simulink model "simulation_part1"  (R2021b)
settings: Solver=VariableStepAuto  StartTime=0.0  StopTime=10.0  RelTol=1e-3
values from neighbouring files (symbols this model uses):
  A = [0.0702214917532  -0.116010526395  -1.08987824045; 0.410067295195  -0.932250543618  -1.24586844105; -0.123091124979  1.5728866522  -0.314709957878]    [ex2_data.mat]
  B1 = [-0.999067654878  0.651260985893; 0.287497412628  0.148151711186; 0.248638319418  2.25662896165]    [ex2_data.mat]
  B2 = [0.722863093118  0.264721524509; 0.0846003934803  0.180309892623; -1.95559499489  1.07897348192]    [ex2_data.mat]
  C1 = [2.31275280612  0.189359533817  1.67949548769; 0.186530271276  1.56272046404  -1.25277472596]    [ex2_data.mat]
  C2 = [-0.336197041449  0.851608289148  0.411251123774; 1.34398190607  0.500911743536  0.482620057996]    [ex2_data.mat]
  D1 = [1  0; 0  1]    [ex2_data.mat]
  K = inv(R)*B2'*P    [ex2.m]
settings Model: Creator=Marius  LastModifiedBy=Marius

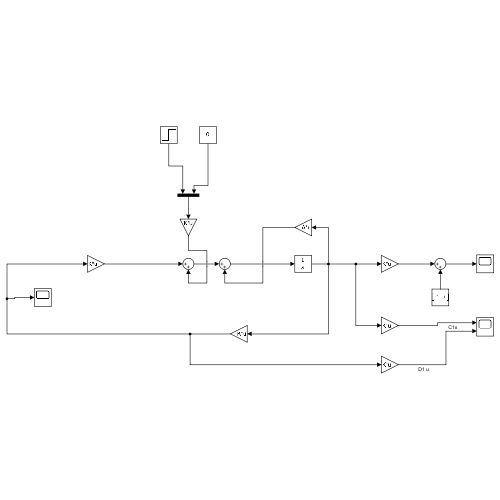
[thumbnail: Simulink's stored preview of the top-level diagram]
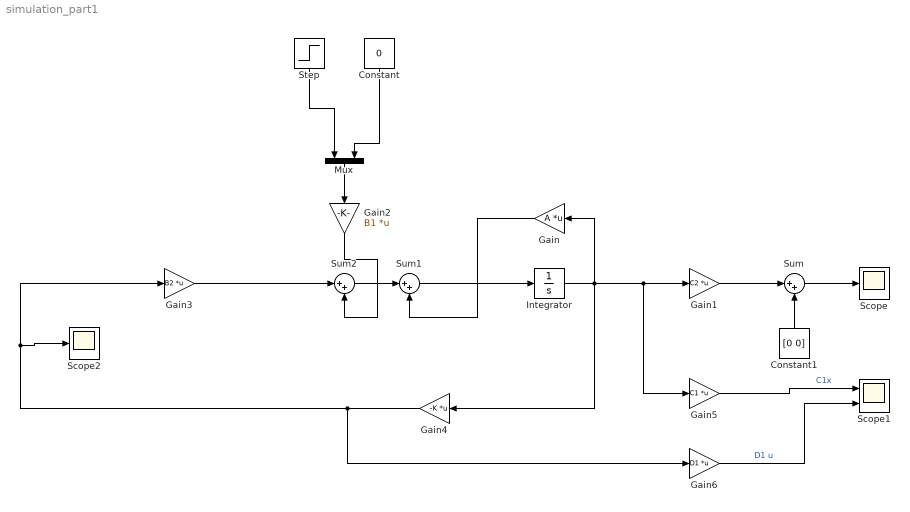
== system simulation_part1 ==
  Constant : Constant  Value=0
  Constant1 : Constant  Value=[0 0]
  Gain : Gain  Gain=A  Multiplication=Matrix(K*u)
  Gain1 : Gain  Gain=C2  Multiplication=Matrix(K*u)
  Gain2 : Gain  Gain=B1  Multiplication=Matrix(K*u)
  Gain3 : Gain  Gain=B2  Multiplication=Matrix(K*u)
  Gain4 : Gain  Gain=-K  Multiplication=Matrix(K*u)
  Gain5 : Gain  Gain=C1  Multiplication=Matrix(K*u)
  Gain6 : Gain  Gain=D1  Multiplication=Matrix(K*u)
  Integrator : Integrator
  Mux : Mux  Inputs=2
  Scope : Scope
  Scope1 : Scope  NumInputPorts=2
  Scope2 : Scope
  Step : Step  SampleTime=0
  Sum : Sum  Inputs=|++
  Sum1 : Sum  Inputs=|++
  Sum2 : Sum  Inputs=|++
  wires:
  Integrator/1 -> Gain4/1, Gain/1, Gain5/1, Gain1/1
  Gain/1 -> Sum1/2
  Sum1/1 -> Integrator/1
  Gain1/1 -> Sum/1
  Gain3/1 -> Sum2/1
  Sum2/1 -> Sum1/1
  Gain2/1 -> Sum2/2
  Sum/1 -> Scope/1
  Constant1/1 -> Sum/2
  Gain4/1 -> Gain6/1, Scope2/1, Gain3/1
  Mux/1 -> Gain2/1
  Step/1 -> Mux/1
  Constant/1 -> Mux/2
  Gain5/1 -> Scope1/1  "C1x"
  Gain6/1 -> Scope1/2  "D1 u"
